simulink model "state_machine"  (R2022a)
settings: Solver=VariableStepAuto  StartTime=0.0  StopTime=10.0  RelTol=1e-3
libraries: SignalEditorBlockLib x1
settings Model: Creator=cc  LastModifiedBy=cc

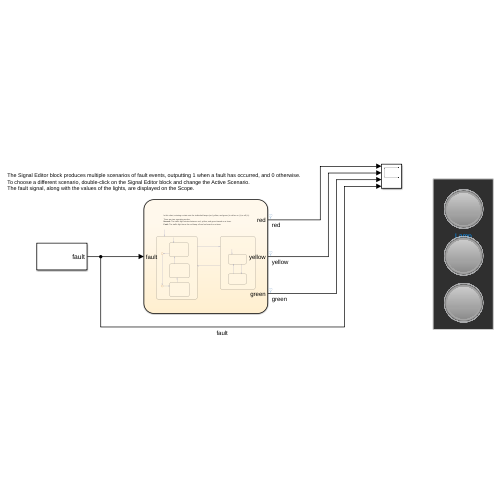
[thumbnail: Simulink's stored preview of the top-level diagram]
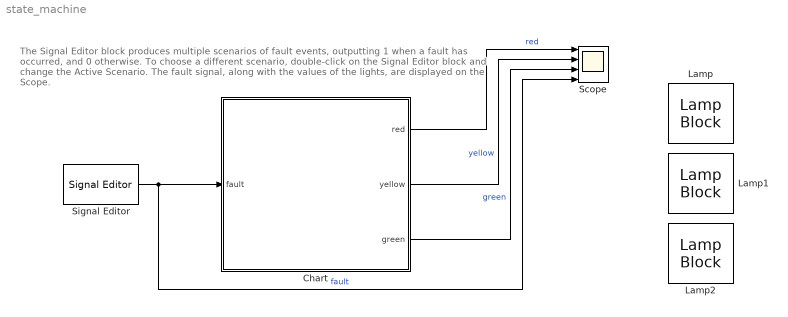
== system state_machine ==
  note: The Signal Editor block produces multiple scenarios of fault events, outputting 1 when a fault has occurred, and 0 otherwise.
      | To choose a different scenario, double-click on the Signal Editor block and change the Active Scenario.
      | The fault signal, along with the values of the lights, are displayed on the Scope.
  Chart : Stateflow chart  TreatAsAtomicUnit=on
  Lamp : LampBlock  LabelPosition=Hide
  Lamp1 : LampBlock  LabelPosition=Hide
  Lamp2 : LampBlock  LabelPosition=Hide
  Scope : Scope  NumInputPorts=4
  Signal Editor : SignalEditorBlockLib/Signal Editor  FileName=trafficLightFault.mat  ActiveScenario=Faults  ActiveSignal=fault  IsBus=off  OutputBusObjectStr=Bus: BusObject  SampleTime=1  Interpolate=off  ZeroCross=off  OutputAfterFinalValue=Setting to zero  Unit=inherit  PreserveSignalName=on
  wires:
  Chart/3(green) -> Scope/3  "green"
  Chart/1(red) -> Scope/1  "red"
  Signal Editor/1 -> Chart/1(fault), Scope/4  "fault"
  Chart/2(yellow) -> Scope/2  "yellow"

== stateflow chart state_machine/Chart ==
  note: In this chart, entering a state sets the individual lamps (red, yellow, and green) to either on ( 1 ) or off ( 0 ).
      |
      | There are two operating modes.
      | Normal: The traffic light rotates between red, yellow, and green based on a timer.
      | Fault: The traffic light turns the red lamp off and on based on a timer.
  state Normal
    state Stop
      % Red light
      entry:
      red = 1;
      yellow = 0;
      green = 0;
    state PrepareToStop
      % Yellow light
      entry:
      red = 0;
      yellow = 1;
      green = 0;
    state Go
      % Green light
      entry:
      red = 0;
      yellow = 0;
      green = 1;
    (default) -> Stop
    Stop -> (junction 26)
    (junction 26) -> (junction 29) : after(3,sec)
    PrepareToStop -> Stop : after(3,sec)
    Go -> PrepareToStop : after(15,sec)
    (junction 29) -> Go
  state Fault
    entry:
    yellow = 0;
    green = 0;
    state BlinkOn
      % Red light
      entry:
      red = 1;
    state BlinkOff
      % No light
      entry:
      red = 0;
    (default) -> BlinkOn
    BlinkOff -> BlinkOn : after(1,sec)
    BlinkOn -> BlinkOff : after(1,sec)
  (default) -> Normal
  Normal -> Fault : [fault == 1]
  Fault -> Normal : [fault == 0]
  data: red output =1; yellow output; fault input; green output =0
